simulink model "app_designer"  (R2018b)
settings: Solver=FixedStepAuto  StartTime=0.0  StopTime=Inf  FixedStep=1  RelTol=1e-3  EnableMultiTasking=on
values from neighbouring files (symbols this model uses):
  cpw = 4175    [app.mat]
  Cv01 = 801600    [app.mat]
  Cv02 = 801600    [app.mat]
  Cvg1 = 400800    [app.mat]
  Cvg2 = 400800    [app.mat]
  Cvs1 = 38412000    [app.mat]
  Cvs2 = 38412000    [app.mat]
  Cvw1 = 60000    [app.mat]
  Cvw2 = 60000    [app.mat]
  dfmw = 0    [app.mat]
  dTwz = 0    [app.mat]
  dTzew = 0    [app.mat]
  fmg1_0 = 0.0239520958084    [app.mat]
  fmg2_0 = 0.0239520958084    [app.mat]
  fmw0 = 0.0479041916168    [app.mat]
  Kcg1 = 40    [app.mat]
  Kcg2 = 40    [app.mat]
  Kco = 200    [app.mat]
  Kcs1 = 80    [app.mat]
  Kcs2 = 80    [app.mat]
  Kcw1 = 133.333333333    [app.mat]
  Kcw2 = 133.333333333    [app.mat]
  steptime = 30000    [app.mat]
  Tdelay1 = 16000    [app.mat]
  Tdelay2 = 16000    [app.mat]
  Tgp1_0 = 70    [app.mat]
  Tgp2_0 = 70    [app.mat]
  Toz0 = 90    [app.mat]
  Ts1_0 = 5    [app.mat]
  Ts2_0 = 5    [app.mat]
  Twew1_0 = 20    [app.mat]
  Twew2_0 = 20    [app.mat]
  Twp0 = 110    [app.mat]
  Twz0 = 130    [app.mat]
  Tzew0 = -20    [app.mat]
Description:
  | Water Tank Model with Dashboard
  | 
  | The example model "sldrtex_dashboard" shows a real-time model of a water tank
  | controlled by dashboard controls.  You can change the inputs to the plant using
  | the knobs and observe the response on the gauges.
  | 
  | How to run this model in Normal Mode:
  | 
  | 1) Double-click the orange button to switch to Normal Mode if needed.
  | 2) Start the real-time execution using Simulation->Run.
  | 3) Change the input flow and output valve values by the dashboard controls and observe
  |    the results on the dashboard gauges.
  | 
  | How to run this model in External Mode:
  | 
  | 1) Double-click the orange button to switch to External Mode if needed.
  | 2) Start the real-time execution using Simulation->Run. The model will automatically
  |    build, connect to Simulink in External Mode and start.
  | 3) Change the input flow and output valve values by the dashboard controls and observe
  |    the results on the dashboard gauges.
settings Model: EnablePacing=on  PacingRate=100000  ExtModeTrigDuration=101  Creator=The MathWorks, Inc.  LastModifiedBy=r3vus
settings Model: SetupFcn=|
  | %The GUI handles are by default hidden, turn them on
  | set(0,'ShowHiddenHandles','on');
  | 
  | %Set up the arguments that will go into the gain block event callback listener
  | blk = 'app_designer/Gain';
  | event = 'PostOutputs';
  | listener = @updateVal;
  | 
  | %Create the listener
  | h = add_exec_event_listener(blk, event, listener);
settings DataIOCC: LimitDataPoints=on  MaxDataPoints=100000  SaveFormat=Array  ReturnWorkspaceOutputs=on  SignalLoggingName=logsOut  LoggingIntervals=[0, 10000]
settings OptimizationCC: ExpressionDepthLimit=2147483647  InitFltsAndDblsToZero=on  EfficientMapNaN2IntZero=off  LifeSpan=inf
settings DebuggingCC: UnderspecifiedInitializationDetection=Classic  MergeDetectMultiDrivingBlocksExec=none  SignalResolutionControl=TryResolveAllWithWarning  FcnCallInpInsideContextMsg=warning  AllowSymbolicDim=off  StateNameClashWarn=warning  SFUnexpectedBacktrackingDiag=warning  SFNoUnconditionalDefaultTransitionDiag=warning  SFExecutionAtInitializationDiag=none
settings HardwareCC: TargetBitPerLong=64  TargetBitPerPointer=64  TargetBitPerSizeT=64  TargetBitPerPtrDiffT=64  TargetIntDivRoundTo=Zero  TargetEndianess=LittleEndian  TargetWordSize=64  TargetHWDeviceType=Intel->x86-64
settings ModelReferenceCC: PropagateSignalLabelsOutOfModel=off
settings SFSimCC: SimUseLocalCustomCode=off
settings RTWCC: SystemTargetFile=sldrt.tlc  TemplateMakefile=sldrt.tmf  Description=Simulink Desktop Real-Time  RTWUseLocalCustomCode=off  RTWCompilerOptimization=on
settings CodeAppCC: MaxIdLength=95  StateflowObjectComments=on
settings SimulinkDesktopRealTimeCC: TargetPreCompLibLocation=D:\MATLAB\R2018b\toolbox\sldrt\lib\win64  TargetLangStandard=C89/C90 (ANSI)  GeneratePreprocessorConditionals=Disable all  SupportVariableSizeSignals=off  PreserveStateflowLocalDataDimensions=off
settings ConfigComp: CovMetricSettings=dw  CovHtmlReporting=on  CovSaveCumulativeToWorkspaceVar=on  CovSaveSingleToWorkspaceVar=on  CovShowResultsExplorer=off  CovExternalEMLEnable=off  CovSFcnEnable=off

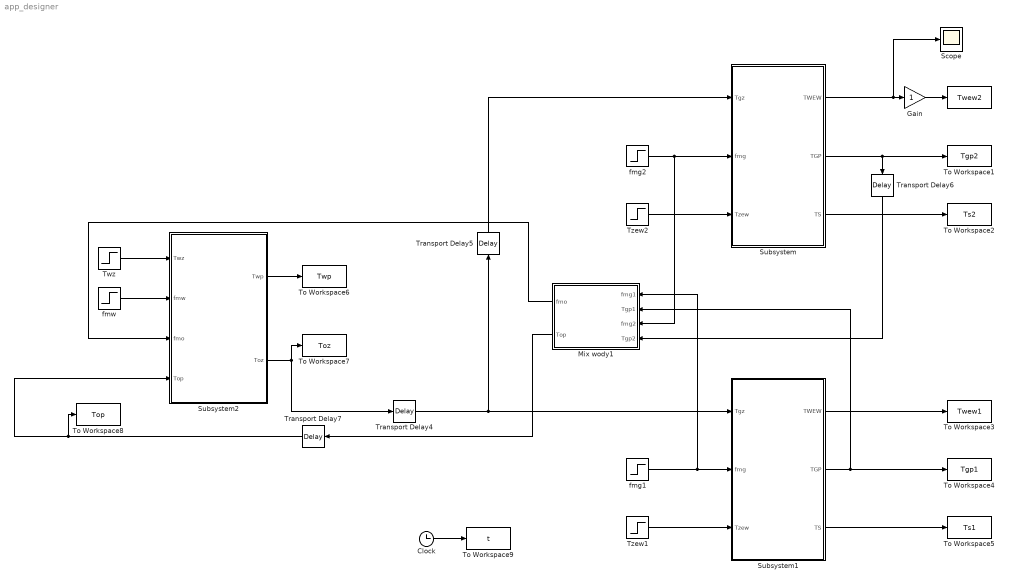
== system app_designer ==
  " " : ToWorkspace  VariableName=Twew2  SaveFormat=Structure With Time  SampleTime=-1
  Clock : Clock
  Gain : Gain
  Mix wody1 : Subsystem
  Scope : Scope
  Subsystem : Subsystem  mask{Cvg=Cvg2, Cvs=Cvs2, Kcg=Kcg2, Kcw=Kcw2, cpw=cpw, Kcs=Kcs2, Cvw=Cvw2, Twew0=Twew2_0, Ts0=Ts2_0, Tgp0=Tgp2_0}
  Subsystem1 : Subsystem  mask{Cvg=Cvg1, Cvs=Cvs1, Kcg=Kcg1, Kcw=Kcw1, cpw=cpw, Kcs=Kcs1, Cvw=Cvw1, Twew0=Twew1_0, Ts0=Ts1_0, Tgp0=Tgp1_0}
  Subsystem2 : Subsystem
  To Workspace1 : ToWorkspace  VariableName=Tgp2  SampleTime=-1
  To Workspace2 : ToWorkspace  VariableName=Ts2  SampleTime=-1
  To Workspace3 : ToWorkspace  VariableName=Twew1  SampleTime=-1
  To Workspace4 : ToWorkspace  VariableName=Tgp1  SampleTime=-1
  To Workspace5 : ToWorkspace  VariableName=Ts1  SampleTime=-1
  To Workspace6 : ToWorkspace  VariableName=Twp  SampleTime=-1
  To Workspace7 : ToWorkspace  VariableName=Toz  SampleTime=-1
  To Workspace8 : ToWorkspace  VariableName=Top  SampleTime=-1
  To Workspace9 : ToWorkspace  VariableName=t  SampleTime=-1
  Transport Delay4 : TransportDelay  DelayTime=Tdelay1  InitialOutput=Toz0
  Transport Delay5 : TransportDelay  DelayTime=Tdelay2  InitialOutput=Toz0
  Transport Delay6 : TransportDelay  DelayTime=Tdelay2  InitialOutput=Tgp2_0
  Transport Delay7 : TransportDelay  DelayTime=Tdelay1  InitialOutput=(Tgp1_0*fmg1_0+Tgp2_0*fmg2_0)/(fmg1_0+fmg2_0)
  Twz : Step  Time=steptime  Before=Twz0  After=Twz0+dTwz  SampleTime=0
  Tzew1 : Step  Time=steptime  Before=Tzew0  After=Tzew0+dTzew  SampleTime=0
  Tzew2 : Step  Time=steptime  Before=Tzew0  After=Tzew0+dTzew  SampleTime=0
  fmg1 : Step  Time=steptime  Before=fmg1_0  After=fmg1_0  SampleTime=0
  fmg2 : Step  Time=steptime  Before=fmg2_0  After=fmg2_0  SampleTime=0
  fmw : Step  Time=steptime  Before=fmw0  After=fmw0+dfmw  SampleTime=0
  wires:
  Clock/1 -> To Workspace9/1
  Transport Delay7/1 -> To Workspace8/1, Subsystem2/4(Top)
  Transport Delay5/1 -> Subsystem/1(Tgz)
  Subsystem/2(TGP) -> Transport Delay6/1, To Workspace1/1
  fmg1/1 -> Mix wody1/1(fmg1), Subsystem1/2(fmg)
  Subsystem2/1(Twp) -> To Workspace6/1
  Tzew1/1 -> Subsystem1/3(Tzew)
  Mix wody1/2(Top) -> Transport Delay7/1
  Subsystem1/2(TGP) -> Mix wody1/2(Tgp1), To Workspace4/1
  fmw/1 -> Subsystem2/2(fmw)
  Subsystem/3(TS) -> To Workspace2/1
  Tzew2/1 -> Subsystem/3(Tzew)
  Subsystem1/1(TWEW) -> To Workspace3/1
  Transport Delay6/1 -> Mix wody1/4(Tgp2)
  Subsystem2/2(Toz) -> Transport Delay4/1, To Workspace7/1
  Subsystem1/3(TS) -> To Workspace5/1
  Twz/1 -> Subsystem2/1(Twz)
  Transport Delay4/1 -> Transport Delay5/1, Subsystem1/1(Tgz)
  Mix wody1/1(fmo) -> Subsystem2/3(fmo)
  fmg2/1 -> Mix wody1/3(fmg2), Subsystem/2(fmg)
  Gain/1 -> " "/1
  Subsystem/1(TWEW) -> Gain/1, Scope/1

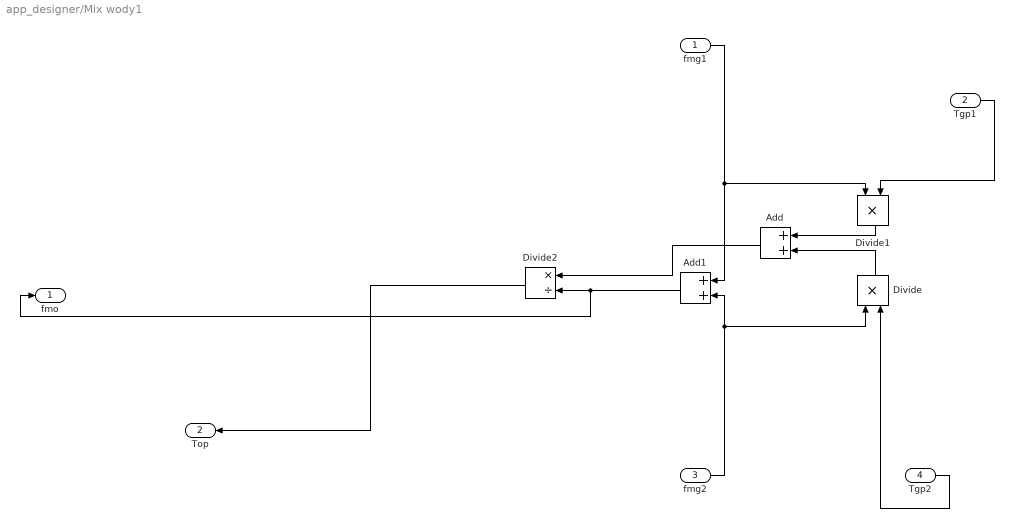
== system app_designer/Mix wody1 ==
  fmg1 : Inport
  Tgp1 : Inport  Port=2
  fmg2 : Inport  Port=3
  Tgp2 : Inport  Port=4
  Add : Sum
  Add1 : Sum
  Divide : Product  Inputs=**
  Divide1 : Product  Inputs=**
  Divide2 : Product  Inputs=*/
  fmo : Outport
  Top : Outport  Port=2
  wires:
  Tgp1/1 -> Divide1/2
  fmg2/1 -> Add1/2, Divide/1
  Divide/1 -> Add/2
  Add1/1 -> fmo/1, Divide2/2
  Tgp2/1 -> Divide/2
  fmg1/1 -> Add1/1, Divide1/1
  Divide1/1 -> Add/1
  Add/1 -> Divide2/1
  Divide2/1 -> Top/1

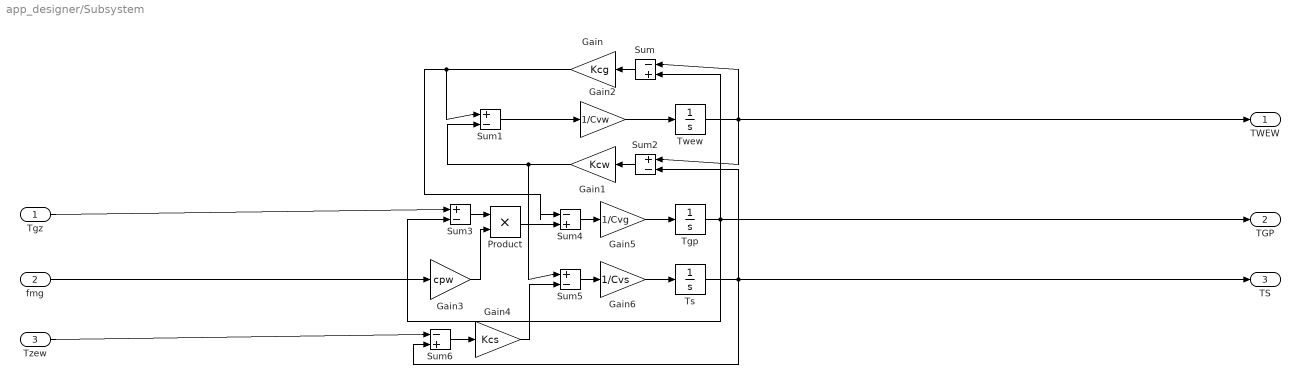
== system app_designer/Subsystem ==
  Tgz : Inport
  fmg : Inport  Port=2
  Tzew : Inport  Port=3
  Gain : Gain  Gain=Kcg
  Gain1 : Gain  Gain=Kcw
  Gain2 : Gain  Gain=1/Cvw
  Gain3 : Gain  Gain=cpw
  Gain4 : Gain  Gain=Kcs
  Gain5 : Gain  Gain=1/Cvg
  Gain6 : Gain  Gain=1/Cvs
  Product : Product
  Sum : Sum  Inputs=|-+
  Sum{1..3,5} (4 alike) : Sum  Inputs=|+-
  Sum4 : Sum  Inputs=|-+
  Sum6 : Sum  Inputs=|-+
  Tgp : Integrator  InitialCondition=Tgp0
  Ts : Integrator  InitialCondition=Ts0
  Twew : Integrator  InitialCondition=Twew0
  TWEW : Outport
  TGP : Outport  Port=2
  TS : Outport  Port=3
  wires:
  Twew/1 -> TWEW/1, Sum2/1, Sum/1
  Tgp/1 -> TGP/1, Sum3/2, Sum/2
  Sum/1 -> Gain/1
  Ts/1 -> TS/1, Sum6/2, Sum2/2
  Sum2/1 -> Gain1/1
  Gain1/1 -> Sum5/1, Sum1/2
  Sum1/1 -> Gain2/1
  Tgz/1 -> Sum3/1
  fmg/1 -> Gain3/1
  Gain3/1 -> Product/2
  Sum3/1 -> Product/1
  Gain/1 -> Sum1/1, Sum4/1
  Product/1 -> Sum4/2
  Sum4/1 -> Gain5/1
  Tzew/1 -> Sum6/1
  Sum6/1 -> Gain4/1
  Gain4/1 -> Sum5/2
  Sum5/1 -> Gain6/1
  Gain2/1 -> Twew/1
  Gain5/1 -> Tgp/1
  Gain6/1 -> Ts/1

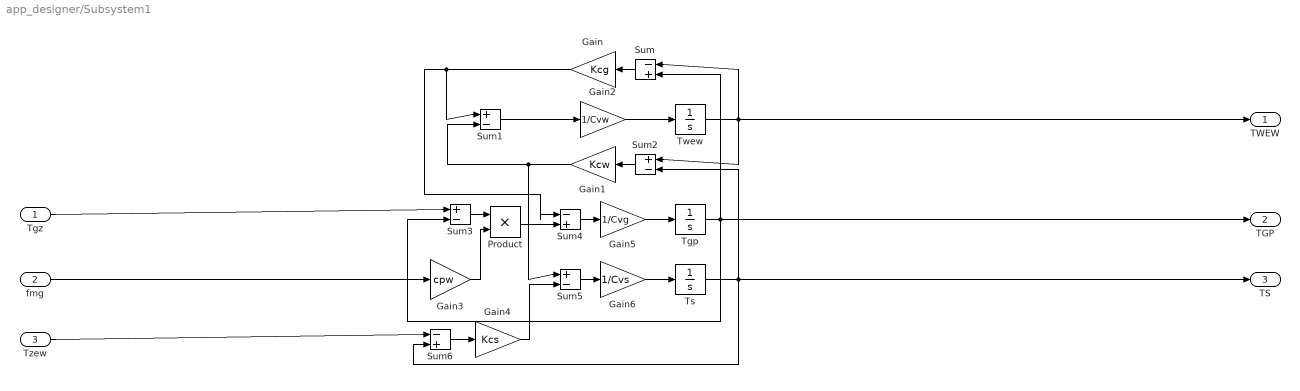
== system app_designer/Subsystem1 ==
  Tgz : Inport
  fmg : Inport  Port=2
  Tzew : Inport  Port=3
  Gain : Gain  Gain=Kcg
  Gain1 : Gain  Gain=Kcw
  Gain2 : Gain  Gain=1/Cvw
  Gain3 : Gain  Gain=cpw
  Gain4 : Gain  Gain=Kcs
  Gain5 : Gain  Gain=1/Cvg
  Gain6 : Gain  Gain=1/Cvs
  Product : Product
  Sum : Sum  Inputs=|-+
  Sum{1..3,5} (4 alike) : Sum  Inputs=|+-
  Sum4 : Sum  Inputs=|-+
  Sum6 : Sum  Inputs=|-+
  Tgp : Integrator  InitialCondition=Tgp0
  Ts : Integrator  InitialCondition=Ts0
  Twew : Integrator  InitialCondition=Twew0
  TWEW : Outport
  TGP : Outport  Port=2
  TS : Outport  Port=3
  wires:
  Twew/1 -> TWEW/1, Sum2/1, Sum/1
  Tgp/1 -> TGP/1, Sum3/2, Sum/2
  Sum/1 -> Gain/1
  Ts/1 -> TS/1, Sum6/2, Sum2/2
  Sum2/1 -> Gain1/1
  Gain1/1 -> Sum5/1, Sum1/2
  Sum1/1 -> Gain2/1
  Tgz/1 -> Sum3/1
  fmg/1 -> Gain3/1
  Gain3/1 -> Product/2
  Sum3/1 -> Product/1
  Gain/1 -> Sum1/1, Sum4/1
  Product/1 -> Sum4/2
  Sum4/1 -> Gain5/1
  Tzew/1 -> Sum6/1
  Sum6/1 -> Gain4/1
  Gain4/1 -> Sum5/2
  Sum5/1 -> Gain6/1
  Gain2/1 -> Twew/1
  Gain5/1 -> Tgp/1
  Gain6/1 -> Ts/1

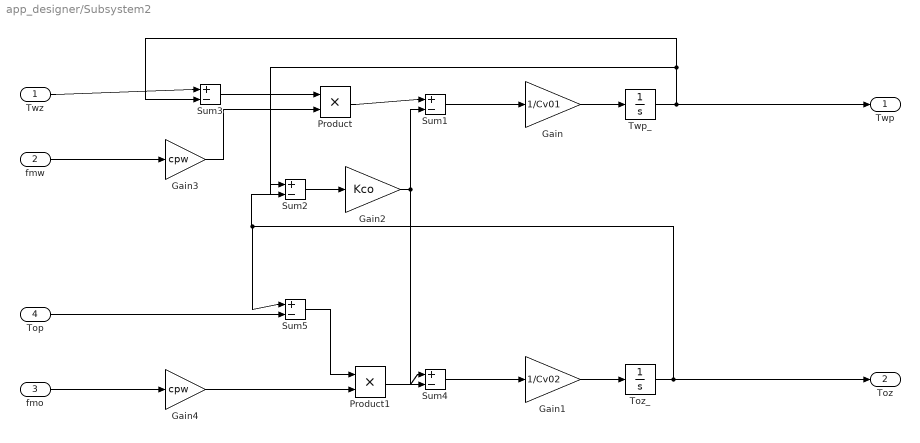
== system app_designer/Subsystem2 ==
  Twz : Inport
  fmw : Inport  Port=2
  fmo : Inport  Port=3
  Top : Inport  Port=4
  Gain : Gain  Gain=1/Cv01
  Gain1 : Gain  Gain=1/Cv02
  Gain2 : Gain  Gain=Kco
  Gain3 : Gain  Gain=cpw
  Gain4 : Gain  Gain=cpw
  Product : Product
  Product1 : Product
  Sum{1..5} (5 alike) : Sum  Inputs=|+-
  Toz_ : Integrator  InitialCondition=Toz0
  Twp_ : Integrator  InitialCondition=Twp0
  Twp : Outport
  Toz : Outport  Port=2
  wires:
  Toz_/1 -> Sum5/1, Sum2/2, Toz/1
  Twp_/1 -> Sum2/1, Sum3/2, Twp/1
  Gain/1 -> Twp_/1
  Gain1/1 -> Toz_/1
  Gain3/1 -> Product/2
  fmw/1 -> Gain3/1
  Sum3/1 -> Product/1
  Twz/1 -> Sum3/1
  Product/1 -> Sum1/1
  Sum1/1 -> Gain/1
  Sum2/1 -> Gain2/1
  Sum4/1 -> Gain1/1
  Gain2/1 -> Sum1/2, Sum4/1
  fmo/1 -> Gain4/1
  Gain4/1 -> Product1/2
  Top/1 -> Sum5/2
  Sum5/1 -> Product1/1
  Product1/1 -> Sum4/2
